simulink model "creating_the_duty_cycle"  (R2024a)
settings: Solver=VariableStepAuto  StartTime=0.0  StopTime=0.0002  RelTol=1e-3
libraries: spsSawtoothGeneratorLib x1, spspowerguiLib x1, spsPWMGeneratorDCDCLib x1
settings Model: Creator=Lenovo  LastModifiedBy=Lenovo

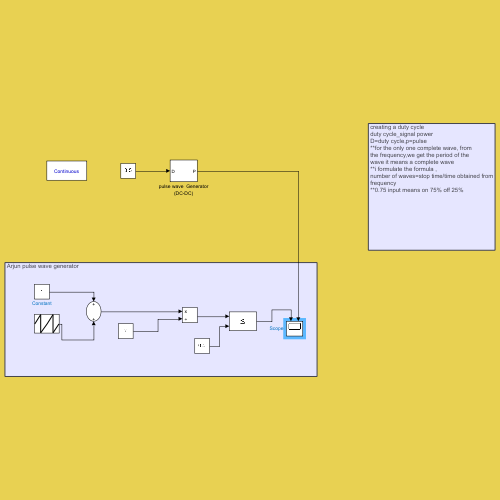
[thumbnail: Simulink's stored preview of the top-level diagram]
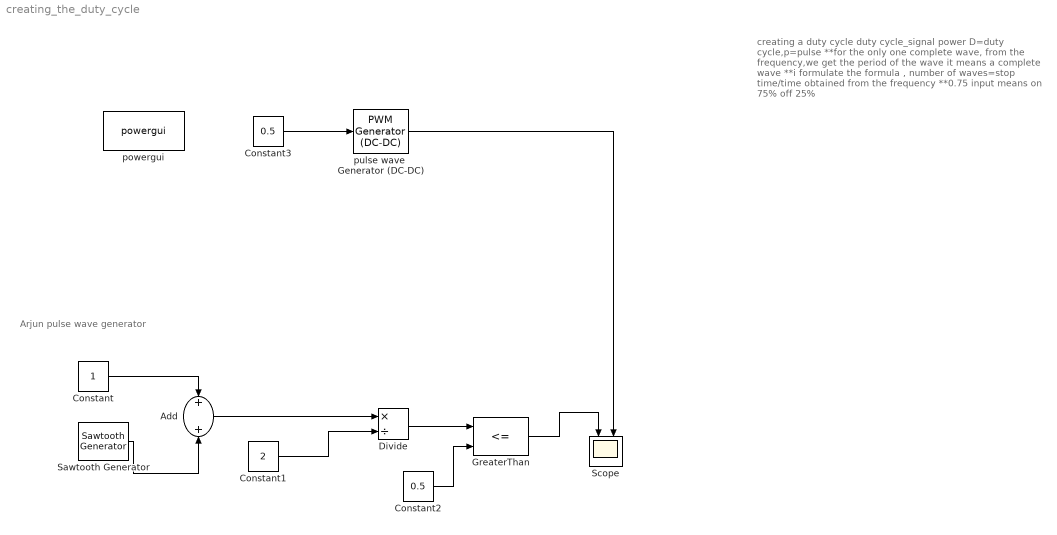
== system creating_the_duty_cycle ==
  note: Arjun pulse wave generator
  note: creating a duty cycle
      | duty cycle_signal power
      | D=duty cycle,p=pulse
      | **for the only one complete wave, from
      | the frequency,we get the period of the
      | wave it means a complete wave
      | **i formulate the formula ,
      | number of waves=stop time/time obtained from the
      | frequency
      | **0.75 input means on 75% off 25%
  Add : Sum
  Constant : Constant
  Constant1 : Constant  Value=2
  Constant2 : Constant  Value=0.5
  Constant3 : Constant  Value=0.5
  Divide : Product  Inputs=*/
  GreaterThan : RelationalOperator  Operator=<=  OutDataTypeStr=boolean  RndMeth=Simplest  InputSameDT=off
  Sawtooth Generator : spsSawtoothGeneratorLib/Sawtooth Generator  Freq=1e4  Phase=180  Ts=0
  Scope : Scope  NumInputPorts=2
  powergui : spspowerguiLib/powergui  Priority=1  SimulationMode=Continuous  SampleTime=50e-6  frequency=60  Iterations=50  frequencyindice=60  Pbase=100e6  ErrMax=1e-4  UnitsV=kV  UnitsW=MW  buscounter=0  FunctionMessages=off  echomessages=off  EnableUseOfTLC=off  CurrentSourceSwitches=off  DisableSnubberDevices=off  DisableRonSwitches=off  DisableVfSwitches=off  DisplayEquations=off  AutomaticDiscreteSolvers=off  SolverType=Tustin/Backward Euler (TBE)  Interpol=off  ExternalGateDelay=off  methode=off  Ts=100  x0status=blocks  SPID=on  SwTol=0  HookPort=off  NonlinearTolerance=1e-4  nMaxIteration=100  ContinueOnMaxIteration=off  RestoreLinks=warning  ResistiveCurrentMeasurement=off  Frange=[0:2:500]  Ylog=off  Xlog=on  ShowGrid=off  save=off  variable=ZData  structure=0  ZoomFFT=off  StartTime=0.0  cycles=1  DisplayStyle=1  fundamental=60  FreqAxis=off  MaxFrequency=1000  frequencyindicesteady=1  RmsSteady=1  display=off
  pulse wave  Generator (DC-DC) : spsPWMGeneratorDCDCLib/PWM Generator (DC-DC)  Fsw=10000  Ts=0
  wires:
  Sawtooth Generator/1 -> Add/2
  Constant/1 -> Add/1
  Add/1 -> Divide/1
  Constant1/1 -> Divide/2
  Constant2/1 -> GreaterThan/2
  Divide/1 -> GreaterThan/1
  GreaterThan/1 -> Scope/1
  Constant3/1 -> pulse wave  Generator (DC-DC)/1
  pulse wave  Generator (DC-DC)/1 -> Scope/2
